simulink model "STRbase_Final_2022"  (R2022a)
settings: Solver=VariableStepAuto  StartTime=0.0  StopTime=10  RelTol=1e-3
settings Model: Creator=user  LastModifiedBy=hakim

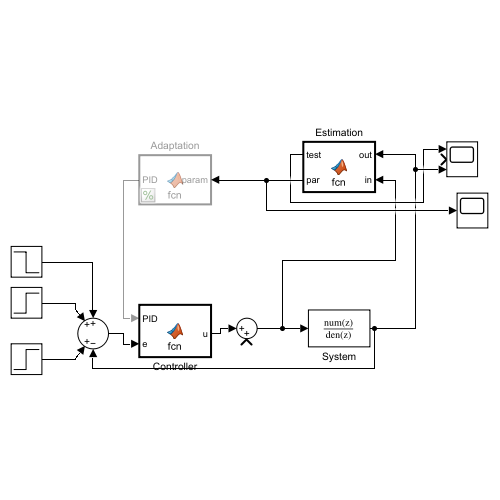
[thumbnail: Simulink's stored preview of the top-level diagram]
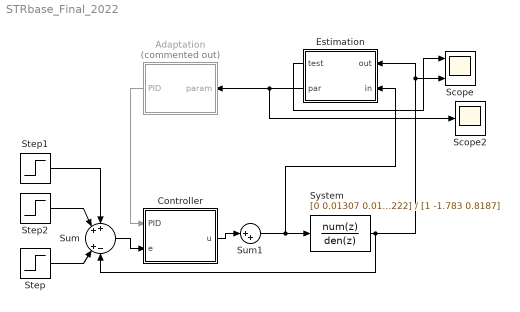
== system STRbase_Final_2022 ==
  Adaptation : MATLAB Function  Commented=on  TreatAsAtomicUnit=on
  Controller : MATLAB Function  TreatAsAtomicUnit=on
  Estimation : MATLAB Function  TreatAsAtomicUnit=on
  Scope : Scope  NumInputPorts=3
  Scope2 : Scope
  Step : Step  Time=50  After=2  SampleTime=0
  Step1 : Step  Time=80  After=-2  SampleTime=0
  Step2 : Step  Time=100  SampleTime=0
  Sum : Sum  Inputs=++||+-
  Sum1 : Sum  Inputs=|++
  System : DiscreteTransferFcn  Numerator=[0 0.01307 0.01222]  Denominator=[1 -1.783 0.8187]  InitialStates=10  SampleTime=0.5
  wires:
  System/1 -> Sum/4, Estimation/1(out), Scope/3
  Estimation/1(test) -> Scope/1
  Sum1/1 -> Estimation/2(in), System/1
  Sum/1 -> Controller/2(e)
  Estimation/2(par) -> Adaptation/1(param), Scope2/1
  Step1/1 -> Sum/1
  Step/1 -> Sum/3
  Step2/1 -> Sum/2
  Controller/1(u) -> Sum1/1
  Adaptation/1(PID) -> Controller/1(PID)

== matlab function STRbase_Final_2022/Controller ==
  data: PID input; u output; e input
function u = fcn(PID, e)
Kp = 1;
Ki = 0;
Kd = 0;

if isempty(PID)
    u = Kp * e + Ki * integral(e) + Kd * diff(e);
else
    [kp, ki, kd] = PID
    u = Kp * e + Ki * integral(e) + Kd * diff(e);
    % Kp = 0.2*Kp+0.8*PID(1);
    % Ki = 0.2*Ki+0.8*PID(2);
    % Kd = 0.2*Kd+0.8*PID(3);


end

== matlab function STRbase_Final_2022/Estimation ==
  data: out input; in input; test output; par output
function [test,par] = fcn(out,in)
%untuk sekarang dibatasin cmn khusus identifikasi dengan orde 2
m=2;
n=2;
lbd=0.97;
persistent ind outd P W 

if isempty(P)
    P=eye(m+n);
end

if isempty(W)
    W=zeros(m+n,1);    
end

if isempty(ind);
    ind=zeros(m,1);
end

if isempty(outd)
    outd=zeros(n,1);
end

%RLS nya
%matrix parameter w mengikuti bentuk x
%x = [y(k-1) y(k-2) u(k-1) u(k-2)]'

%param w kalau di transfer function penjelasan ada di function block
%Adaptation
    x = [outd;ind];
    phi = P*x;
    g = phi/(lbd+x'*phi);
    o = W;
    y= o'*x;
    e = out-y
    W= W+g*e;
    P = (P-g*x'*P)/lbd;

outd=[out;outd(1:1:end-1,:)];
ind=[in;ind(1:1:end-1,:)];

par=W;

%test output variabel apa aja, default nya output RLS yaitu y
test=y;

end

== matlab function STRbase_Final_2022/Adaptation ==
  data: param input; PID output
function PID = fcn(param)
%parameternya ini dibagi jadi dua part
%anggap sistem diskrit dengan 
%NUM = [0 b1 b2]
%DEN = [1 a1 a2]

%param(1) itu koef -y(k-1) atau klo di DEN itu -a1 
%param(2) itu koef -y(k-2) atau klo di DEN itu -a2

%param(3) itu koef u(k-1) atau klo di DEN itu b1 
%param(4) itu koef u(k-2) atau klo di DEN itu b2

a1 = -param(1)
a2 = -param(2)
b1 = param(3)
b2 = param(4)

num = [0 b1 b2]
den = [1 a1 a2]
Tf = tf(num,den)

% [kc,pm,wc,wm] = margin(Tf)
% pu = 2*pi/wc

%PID Parameter

[C] = pidtune(Tf, 'PID')
[kp, ki, kd] = piddata(C)

% kp = kc*0.59;
% ti = pu*0.5;
% td = pu*0.12;
% ki = kp/ti;
% kd = kp*td;

end
